simulink model "BLOCK_Nonlinear_alg_transform_6T"  (R2016b)
settings: Solver=ode15s  StartTime=0.0  StopTime=120  FixedStep=0.01  RelTol=0.01  AbsTol=0.01
settings Model: Creator=Utente  LastModifiedBy=liana
settings SolverCC: MaxOrder=3  MaxConsecutiveMinStep=5  SolverJacobianMethodControl=FullAnalytical  ZeroCrossControl=DisableAll  SolverResetMethod=Robust
settings DataIOCC: SaveState=on
settings OptimizationCC: BlockReduction=off  DefaultParameterBehavior=Inlined  BufferReuse=off

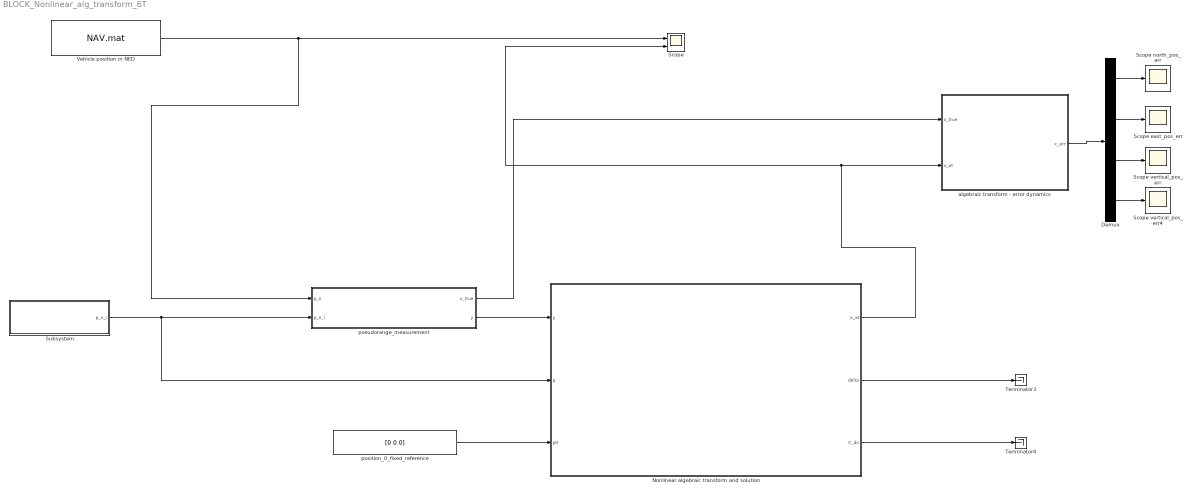
== system BLOCK_Nonlinear_alg_transform_6T ==
  Demux : Demux
  Nonlinear algebraic transform and solution : Subsystem
  Scope : Scope  NumInputPorts=2
  Scope east_pos_err : Scope
  Scope north_pos_err : Scope
  Scope vertical_pos_err : Scope
  Scope vertical_pos_err4 : Scope
  Subsystem : Subsystem
  Terminator3 : Terminator
  Terminator4 : Terminator
  Vehicle position in NED : FromFile  FileName=NAV.mat
  algebraic transform - error dynamics : Subsystem
  position_0_fixed_reference : Constant  Value=[0 0 0]
  "pseudorange_measurement " : Subsystem
  wires:
  Demux/1 -> Scope north_pos_err/1
  Demux/2 -> Scope east_pos_err/1
  Demux/3 -> Scope vertical_pos_err/1
  Nonlinear algebraic transform and solution/1(x_at) -> Scope/2, algebraic transform - error dynamics/2(x_at)
  Demux/4 -> Scope vertical_pos_err4/1
  position_0_fixed_reference/1 -> Nonlinear algebraic transform and solution/3(p0)
  Nonlinear algebraic transform and solution/2(delta) -> Terminator3/1
  Nonlinear algebraic transform and solution/3(C_dx) -> Terminator4/1
  Vehicle position in NED/1 -> "pseudorange_measurement "/1(p_n), Scope/1
  "pseudorange_measurement "/2("y ") -> Nonlinear algebraic transform and solution/1(y)
  algebraic transform - error dynamics/1(x_err) -> Demux/1
  "pseudorange_measurement "/1(x_true) -> algebraic transform - error dynamics/1(x_true)
  Subsystem/1(p_n_i) -> Nonlinear algebraic transform and solution/2(p), "pseudorange_measurement "/2(p_n_i)

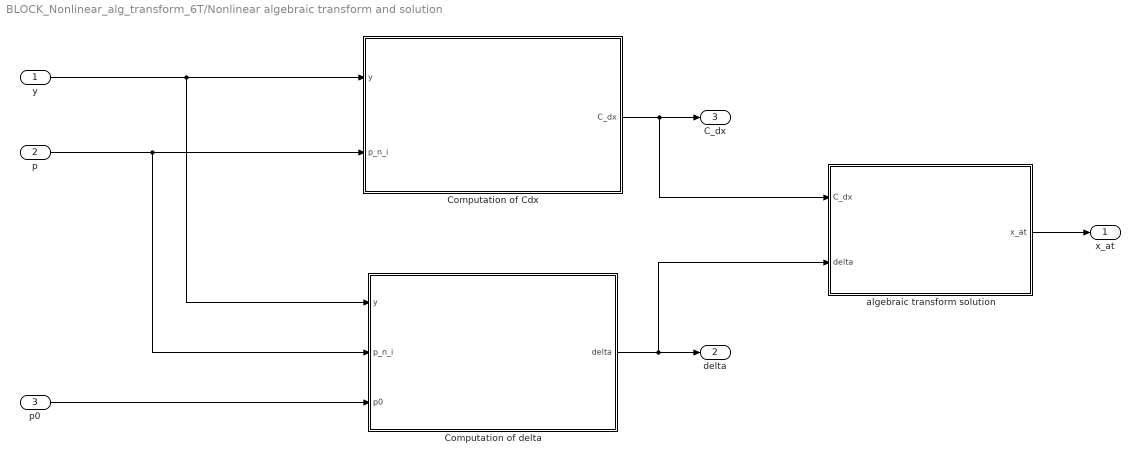
== system BLOCK_Nonlinear_alg_transform_6T/Nonlinear algebraic transform and solution ==
  y : Inport
  p : Inport  Port=2
  p0 : Inport  Port=3
  Computation of Cdx : MATLAB Function  TreatAsAtomicUnit=on
  Computation of delta : MATLAB Function  TreatAsAtomicUnit=on
  algebraic transform solution : MATLAB Function  TreatAsAtomicUnit=on
  x_at : Outport
  delta : Outport  Port=2
  C_dx : Outport  Port=3
  wires:
  y/1 -> Computation of delta/1(y), Computation of Cdx/1(y)
  p/1 -> Computation of delta/2(p_n_i), Computation of Cdx/2(p_n_i)
  p0/1 -> Computation of delta/3(p0)
  Computation of delta/1(delta) -> algebraic transform solution/2(delta), delta/1
  Computation of Cdx/1(C_dx) -> algebraic transform solution/1(C_dx), C_dx/1
  algebraic transform solution/1(x_at) -> x_at/1

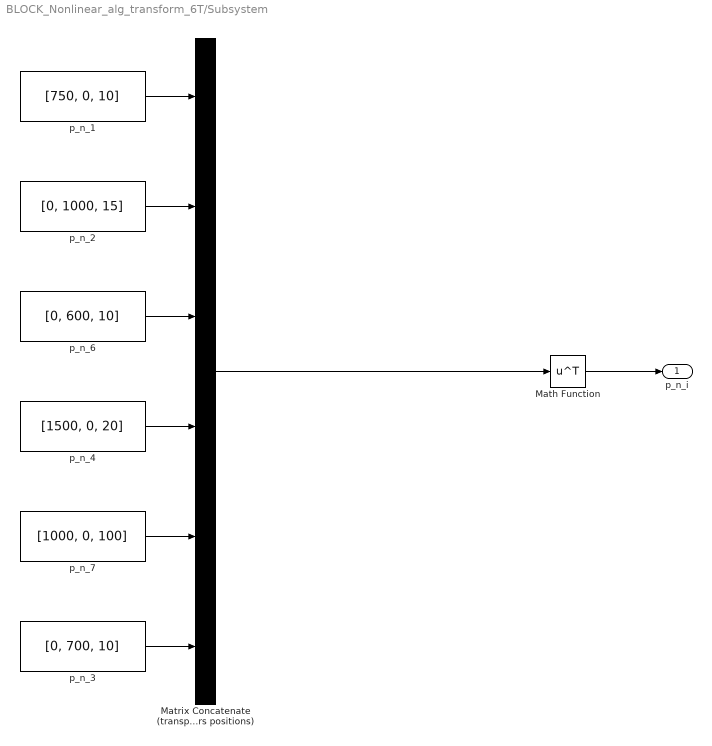
== system BLOCK_Nonlinear_alg_transform_6T/Subsystem ==
  Math Function : Math  Operator=transpose  SaturateOnIntegerOverflow=on
  Matrix Concatenate (transponders positions) : Concatenate  NumInputs=6  Mode=Multidimensional array  ConcatenateDimension=2
  p_n_1 : Constant  Value=[750, 0, 10]
  p_n_2 : Constant  Value=[0, 1000, 15]
  p_n_3 : Constant  Value=[0, 700, 10]
  p_n_4 : Constant  Value=[1500, 0, 20]
  p_n_6 : Constant  Value=[0, 600, 10]
  p_n_7 : Constant  Value=[1000, 0, 100]
  p_n_i : Outport
  wires:
  Matrix Concatenate (transponders positions)/1 -> Math Function/1
  p_n_4/1 -> Matrix Concatenate (transponders positions)/4
  p_n_7/1 -> Matrix Concatenate (transponders positions)/5
  p_n_3/1 -> Matrix Concatenate (transponders positions)/6
  Math Function/1 -> p_n_i/1
  p_n_1/1 -> Matrix Concatenate (transponders positions)/1
  p_n_2/1 -> Matrix Concatenate (transponders positions)/2
  p_n_6/1 -> Matrix Concatenate (transponders positions)/3

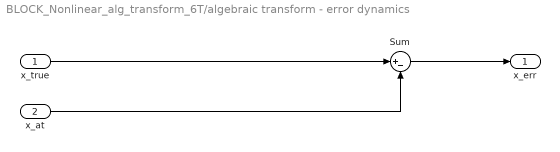
== system BLOCK_Nonlinear_alg_transform_6T/algebraic transform - error dynamics ==
  x_true : Inport
  x_at : Inport  Port=2
  Sum : Sum  Inputs=|+-
  x_err : Outport
  wires:
  x_at/1 -> Sum/2
  Sum/1 -> x_err/1
  x_true/1 -> Sum/1

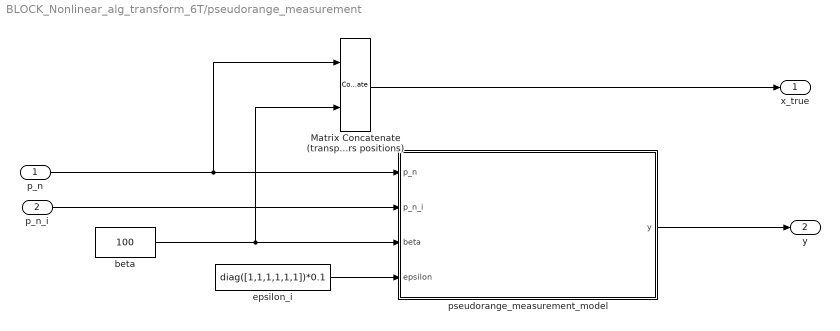
== system BLOCK_Nonlinear_alg_transform_6T/pseudorange_measurement  ==
  p_n : Inport
  p_n_i : Inport  Port=2
  Matrix Concatenate (transponders positions) : Concatenate  Mode=Multidimensional array
  beta : Constant  Value=100
  epsilon_i : Constant  Value=diag([1,1,1,1,1,1])*0.1
  pseudorange_measurement_model : MATLAB Function  TreatAsAtomicUnit=on
  x_true : Outport
  "y " : Outport  Port=2
  wires:
  p_n_i/1 -> pseudorange_measurement_model/2(p_n_i)
  pseudorange_measurement_model/1(y) -> "y "/1
  epsilon_i/1 -> pseudorange_measurement_model/4(epsilon)
  beta/1 -> Matrix Concatenate (transponders positions)/2, pseudorange_measurement_model/3(beta)
  p_n/1 -> Matrix Concatenate (transponders positions)/1, pseudorange_measurement_model/1(p_n)
  Matrix Concatenate (transponders positions)/1 -> x_true/1

== matlab function BLOCK_Nonlinear_alg_transform_6T/Nonlinear algebraic transform and solution/Computation of Cdx ==
  data: y input; p_n_i input; C_dx output
function C_dx  = C_dx_func(y,p_n_i)

    % y vector 
    % p matrix has row vectors
    %            (x,y,z) cols 
    %            m-rows are transponders number
    % all variables are in navigation frame oh yeah! baby ;)
    
    [row,col] = size(p_n_i);
    [row_,col_] = size(y);
    
    % m-measure vector
    p_m = p_n_i(row,:); % measure of m-th transponder
    y_m = y(row_);  % m-th pseudorange measure

    m = row; % m is transpoders number
    
    
    p_ = zeros(m-1,3); %row vector, 3 stands for x,y,z
    y_ = zeros(m-1,1);
    
    for i = 1 : 1 : m-1
    
        p_(i,:) = p_m - p_n_i(i,:);
        y_(i) = y(i) - y_m;
        
    end
    
    C_dx = [p_, y_];

end

== matlab function BLOCK_Nonlinear_alg_transform_6T/Nonlinear algebraic transform and solution/Computation of delta ==
  data: y input; delta output; p_n_i input; p0 input
function delta   = delta_func(y, p_n_i, p0)

    % y vector 
    % p matrix has row vectors
    %            (x,y,z) cols 
    %            m-rows are the numbers of the transponders
    % all variables are in navigation frame oh yeah! baby ;)
    % z is a col vector of scalars
    
    % we must choose p0 (a block)
    
    [row,col] = size(p_n_i);
    %[row_,col_] = size(y);
    
    p_los = zeros(row,col);
    z = zeros(row,1);   % dim = m x 1
    
    %defining los vector
    for i = 1:1:row
       p_los(i,:) = p_n_i(i,:) - p0';       % dim = m x 3
    end
    
%     p_n_true = p_los;
    
    % p_los = p_los';
    
    for i = 1:1:row
        z(i)= ((y(i)^2) - norm(p_los(i,:))^2); % dim = m x 1
    end
    
%     z = z';
%     
%     delta = zeros(row-1,1);
%     z_m = z(end);
%     
%     for i = 1:1:row-1
%         delta(i) =  (z(i) - z_m); %amm fenito
%     end

    delta = zeros(row-1,1); %dim = (m-1) x 1
    z_m = z(row,1);
    
    for i=1:1:(row-1)
        delta(i,1) = z(i,1) - z_m;
    end

end

== matlab function BLOCK_Nonlinear_alg_transform_6T/pseudorange_measurement /pseudorange_measurement_model ==
  data: p_n input; y output; p_n_i input; beta input; epsilon input
function y = pseudorange_mea_model(p_n, p_n_i, beta, epsilon)

  %  row-vector

  y = zeros(size(p_n_i,1),1);

  for i = 1:1:size(p_n_i,1)

      rho = norm(p_n - (p_n_i(i,:))');  % eq. 7
      
      y(i) = rho + beta + epsilon(i); % eq. 8 

  end
      
end

== matlab function BLOCK_Nonlinear_alg_transform_6T/Nonlinear algebraic transform and solution/algebraic transform solution ==
  data: C_dx input; x_at output; delta input
function x_at = solAT(C_dx, delta)

% this solution is described in the Appendix
% that is correct only for m >= 5

pC_dx = pinv(C_dx);

x_at = pC_dx * (delta / 2);

end
